simulink model "LKAS_AutoSave_20210315_1628"  (R2018b)
settings: Solver=FixedStepDiscrete  StartTime=0.0  StopTime=10.0  FixedStep=0.01  RelTol=1e-3
InitFcn:
  | tmpVer = ver('MATLAB');
  | tmpVer = str2num(tmpVer.Version);
  | % -------------------------------------------------------------------
  | %  MATLAB file generated by Simulink.saveVars on 21-Nov-2019 10:06:14
  | %  MATLAB version: 7.13.0.564 (R2011b)
  | % -------------------------------------------------------------------
  | 
  | 
  | SInt16 = Simulink.AliasType;
  | SInt16.Description = 'Num';
  | if (tmpVer > 7.11)
  | 	SInt16.DataScope = 'Auto';
  | end
  | SInt16.HeaderFile = 'Rte_Type.h';
  | SInt16.BaseType = 'int16';
  | 
  | SInt32 = Simulink.AliasType;
  | SInt32.Description = 'Num';
  | if (tmpVer > 7.11)
  | 	SInt32.DataScope = 'Auto';
  | end
  | SInt32.HeaderFile = 'Rte_Type.h';
  | SInt32.BaseType = 'int32';
  | 
  | SInt8 = Simulink.AliasType;
  | SInt8.Description = 'Num';
  | if (tmpVer > 7.11)
  | 	SInt8.DataScope = 'Auto';
  | end
  | SInt8.HeaderFile = 'Rte_Type.h';
  | SInt8.BaseType = 'int8';
  | 
  | T_A_m2_1024_1_u32 = Simulink.NumericType;
  | T_A_m2_1024_1_u32.Description = 'm2 (square meters  (m2))';
  | if (tmpVer > 7.11)
  | 	T_A_m2_1024_1_u32.DataScope = 'Auto';
  | end
  | T_A_m2_1024_1_u32.HeaderFile = 'Rte_Type.h';
  | T_A_m2_1024_1_u32.DataTypeMode = 'Fixed-point: slope and bias scaling';
  | T_A_m2_1024_1_u32.SignednessBool = false;
  | T_A_m2_1024_1_u32.WordLength = 32;
  | T_A_m2_1024_1_u32.FixedExponent = -10;
  | T_A_m2_1024_1_u32.SlopeAdjustmentFactor = 1;
  | T_A_m2_1024_1_u32.Bias = 0;
  | T_A_m2_1024_1_u32.DataTypeOverride = 'Inherit';
  | T_A_m2_1024_1_u32.IsAlias = true;
  | 
  | T_A_m2_65536_1_u16 = Simulink.NumericType;
  | T_A_m2_65536_1_u16.Description = 'm2 (square meters  (m2))';
  | if (tmpVer > 7.11)
  | 	T_A_m2_65536_1_u16.DataScope = 'Auto';
  | end
  | T_A_m2_65536_1_u16.HeaderFile = 'Rte_Type.h';
  | T_A_m2_65536_1_u16.DataTypeMode = 'Fixed-point: slope and bias scaling';
  | T_A_m2_65536_1_u16.SignednessBool = false;
  | T_A_m2_65536_1_u16.WordLength = 16;
  | T_A_m2_65536_1_u16.FixedExponent = -16;
  | T_A_m2_65536_1_u16.SlopeAdjustmentFactor = 1;
  | T_A_m2_65536_1_u16.Bias = 0;
  | T_A_m2_65536_1_u16.DataTypeOverride = 'Inherit';
  | ... (+4598 lines)
StopFcn:
  | clear  T_A_m2_1024_1_u32 T_A_m2_65536_1_u16 T_A_m2_Float32 T_A_mm2_10_1_u16 T_A_mm2_4_1_s16 T_A_mm2_Float32 T_Cnt_Num_10_1_u32 T_Cnt_Num_1_1_s16 T_Cnt_Num_1_1_s32 T_Cnt_Num_1_1_s8 T_Cnt_Num_1_1_u16 T_Cnt_Num_1_1_u32 T_Cnt_Num_1_1_u8 T_E_J_1_1_s32 T_E_J_Float32 T_E_kJ_128_1_s32 T_E_kJ_Float32 T_E_kwh_10_1_u16 T_E_kwh_Float32 T_Epl_kwhpkm_100_1_u16 T_Epl_kwhpkm_Float32 T_F_N_1_1_s16 T_F_N_Float32 T_I_A_1000_1_u16 T_I_A_1048576_1_s32 T_I_A_2048_1_s16 T_I_A_32_1_s16 T_I_A_Float32 T_I_mA_1_1_s16 T_I_mA_32768_128_s16 T_I_mA_Float32 T_J_kgpm2_128_1_u16 T_J_kgpm2_Float32 T_K_NA_1000_1_s16 T_K_NA_100_1_s16 T_K_NA_100_1_u16 T_K_NA_1024_1_s16 T_K_NA_1024_1_u16 T_K_NA_128_1_s16 T_K_NA_128_1_u16 T_K_NA_128_1_u8 T_K_NA_16777216_1_u32 T_K_NA_16_1_s16 T_K_NA_16_1_u16 T_K_NA_16_1_u8 T_K_NA_1_16_u16 T_K_NA_1_1_s16 T_K_NA_1_1_u16 T_K_NA_1_1_u8 T_K_NA_32768_1_s16 T_K_NA_32768_1_u16 T_K_NA_32_1_s8 T_K_NA_4096_1_u16 T_K_NA_4194304_1_s32 T_K_NA_4194304_1_u16 T_K_NA_65536_1_s32 T_K_NA_65536_1_u16 T_K_NA_8192_1_s16 T_K_NA_8_1_s16 T_K_NA_Float32 T_M_Nm_16_1_s16 T_M_Nm_1_1_s16 T_M_Nm_32768_1_s16 T_M_Nm_32_1_s16 T_M_Nm_4_1_s16 T_M_Nm_512_1_s16 T_M_Nm_Float32 T_P_W_1_4_s16 T_P_W_1_8_s16 T_P_W_Float32 T_P_kW_128_1_s16 T_P_kW_1_8_s16 T_P_kW_8_1_s32 T_P_kW_Float32 T_Pct_pct_1024_1_s32 T_Pct_pct_1024_1_u32 T_Pct_pct_10_1_s16 T_Pct_pct_10_1_u32 T_Pct_pct_128_100_s8 T_Pct_pct_1_1_s16 T_Pct_pct_1_4_u8 T_Pct_pct_255_100_u16 T_Pct_pct_255_100_u8 T_Pct_pct_256_1_s16 T_Pct_pct_256_1_u16 T_Pct_pct_65535_100_u16 T_Pct_pct_Float32 T_R_ohm_1024_1_s16 T_R_ohm_32_1_s16 T_R_ohm_Float32 T_TK_K_16_1_s16 T_TK_K_Float32 T_T_degC_10_400_1_u16 T_T_degC_16_1_s16 T_T_degC_1_40_1_u8 T_T_degC_2_80_1_u8 T_T_degC_Float32 T_U_V_1000_1_u16 T_U_V_10_1_u8 T_U_V_200_1_u8 T_U_V_32_1_s16 T_U_V_4096_1_s16 T_U_V_512_1_s16 T_U_V_65535_8_u16 T_U_V_8192_1_u16 T_U_V_Float32 T_U_mV_1_1_s16 T_U_mV_256_20_u16 T_U_mV_Float32 T_V_l_256_1_s16 T_V_l_4096_1_s16 T_V_l_64_1_s16 T_V_l_65535_100_u16 T_V_l_Float32 T_V_ml_128_1_s16 T_V_ml_1_1_s16 T_V_ml_32768_1_s16 T_V_ml_Float32 T_V_ul_32_1_u16 T_V_ul_Float32 T_Vpl_clpkm_512_1_u16 T_Vpl_clpkm_Float32 T_a_kphps_16_1_s16 T_a_kphps_Float32 T_a_mps2_128_1_s16 T_a_mps2_Float32 T_c_MJpkg_256_1_s16 T_c_MJpkg_Float32 T_c_kJpgpK_1024_1_s16 T_c_kJpgpK_Float32 T_c_kJpkgpK_128_1_u16 T_c_kJpkgpK_Float32 T_chrg_Ah_1_1_s16 T_chrg_Ah_1_1_u16 T_chrg_Ah_1_1_u8 T_chrg_Ah_256_1_u16 T_chrg_Ah_4194304_1_s32 T_chrg_Ah_512_1_u16 T_chrg_Ah_8_1_u16 T_chrg_Ah_Float32 T_cmp_NA_100_1_s16 T_cmp_NA_128_1_s16 T_cmp_NA_16_1_s16 T_cmp_NA_32768_1_u16 T_cmp_NA_Float32 T_d2n_rpmps2_4_1_s16 T_d2n_rpmps2_Float32 T_dPct_pctps_16_1_s16 T_dPct_pctps_256_1_s16 T_dPct_pctps_Float32 T_dT_degCps_128_1_s16 T_dT_degCps_Float32 T_dV_lph_1_1_s16 T_dV_lph_Float32 T_dV_lpm_128_1_s16 T_dV_lpm_32_1_s16 T_dV_lpm_Float32 T_dV_lps_1024_1_u16 T_dV_lps_4_1_u16 T_dV_lps_Float32 T_dV_mlps_1024_1_s16 T_dV_mlps_Float32 T_d_BitField16 T_dm_gps_128_1_s16 T_dm_gps_128_1_u16 T_dm_gps_256_1_u16 T_dm_gps_Float32 T_dm_mgps_1_1_s16 T_dm_mgps_Float32 T_dn_rpmps_1_1_s16 T_dn_rpmps_2_1_s16 T_dn_rpmps_Float32 T_dp_Paps_1_1_s16 T_dp_Paps_Float32 T_dp_kPaps_1_1_s16 T_dp_kPaps_8_1_s16 T_dp_kPaps_Float32 T_dphi_degps_128_1_s16 T_dphi_degps_8_1_s16 T_dphi_degps_Float32 T_dr_ps_256_1_s16 T_dr_ps_Float32 T_drho_mgplps_1_2_s16 T_drho_mgplps_Float32 T_e_NA_1_1_u8 T_f_Hz_1_1_u16 T_f_Hz_1_1_u32 T_f_Hz_64_1_u16 T_f_Hz_8_1_s16 T_f_Hz_Float32 T_g_BitField32 T_l_km_16_1_s16 T_l_km_1_1_u16 T_l_km_1_1_u32 T_l_km_Float32 T_l_m_1024_1_s16 T_l_m_16_1_s16 T_l_m_1_1_u32 T_l_m_Float32 T_l_mm_16_1_s16 T_l_mm_1_1_u16 T_l_mm_4096_1_s16 T_l_mm_4_1_u8 T_l_mm_64_1_s16 T_l_mm_Float32 T_m_g_1_1_s16 T_m_g_2048_1_s16 T_m_g_32_1_u16 T_m_g_Float32 T_m_kg_1024_1_s16 T_m_kg_1_1_s16 T_m_kg_1_1_u32 T_m_kg_Float32 T_m_mg_128_1_s16 T_m_mg_32_1_s16 T_m_mg_Float32 T_n_rpm_1_1_s16 T_n_rpm_1_25_u8 T_n_rpm_256_50_u16 T_n_rpm_2_25_u8 T_n_rpm_4_1_u16 T_n_rpm_Float32 T_p_MPa_64_1_s16 T_p_MPa_Float32 T_p_Pa_1_1_s16 T_p_Pa_Float32 T_p_kPa_1_10_u16 T_p_kPa_1_1_s16 T_p_kPa_1_1_u8 T_p_kPa_256_1_u16 T_p_kPa_32_1_u16 T_p_kPa_64_1_s16 T_p_kPa_Float32 T_phi_deg_100_1_s16 T_phi_deg_1024_1_s16 T_phi_deg_128_1_s16 T_phi_deg_1_1_u8 T_phi_deg_256_1_s16 T_phi_deg_2_1_s8 T_phi_deg_32_1_s16 T_phi_deg_512_6_s32 T_phi_deg_Float32 T_phi_rad_2048_1_s16 T_phi_rad_Float32 T_r_NA_1024_1_s16 T_r_NA_1024_1_u16 T_r_NA_16384_1_s16 T_r_NA_16_1_s16 T_r_NA_256_1_s8 T_r_NA_256_1_u16 T_r_NA_32768_1_u16 T_r_NA_32_1_u16 T_r_NA_4096_1_s16 T_r_NA_65535_2_u16 T_r_NA_8192_1_u16 T_r_NA_Float32 T_rho_gpl_8192_1_s16 T_rho_gpl_Float32 T_rho_kgpm3_16_1_s16 T_rho_kgpm3_Float32 T_rho_mgpl_1_1_s16 T_rho_mgpl_64_1_s16 T_rho_mgpl_Float32 T_t_hour_1_1_s16 T_t_hour_Float32 T_t_m_1_1_u16 T_t_m_Float32 T_t_ms_1_1_s16 T_t_ms_1_1_u16 T_t_ms_1_1_u32 T_t_ms_4096_1_s16 T_t_ms_64_1_s16 T_t_ms_Float32 T_t_s_1000_1_s16 T_t_s_100_1_s16 T_t_s_10_1_s16 T_t_s_10_1_u16 T_t_s_1_1_s16 T_t_s_1_1_u16 T_t_s_1_1_u32 T_t_s_Float32 T_t_us_10_1_u32 T_t_us_1_1_s16 T_t_us_1_1_u32 T_t_us_1_4_u16 T_t_us_Float32 T_v_kph_1_1_u8 T_v_kph_64_1_s16 T_v_kph_64_1_u16 T_v_kph_Float32 T_v_mps_256_1_s16 T_v_mps_Float32 T_w_radps_32_1_s16 T_w_radps_Float32 T_y_BitField8 T_y_BitFieldDiagProgress T_y_BitFieldDiagStatus T_y_NA_1_1_u8 SInt16 SInt32 SInt8 T_BOOLEAN UInt16 UInt32 UInt8 s16 s32 s8 u16 u32 u8
model workspace (MAT data in the model file):
  MCOS : class17 (value not decoded)
  MCOS : class17 (value not decoded)
  MCOS : class17 (value not decoded)
  MCOS : class17 (value not decoded)
  MCOS : class17 (value not decoded)
  MCOS : class17 (value not decoded)
  MCOS : class17 (value not decoded)
  MCOS : class17 (value not decoded)
  MCOS : class17 (value not decoded)
  MCOS : class17 (value not decoded)
  MCOS : class17 (value not decoded)
  MCOS : class17 (value not decoded)
  MCOS : class17 (value not decoded)
  MCOS : class17 (value not decoded)
  MCOS : class17 (value not decoded)
  MCOS : class17 (value not decoded)
  MCOS : class17 (value not decoded)
  MCOS : class17 (value not decoded)
  MCOS : class17 (value not decoded)
  MCOS : class17 (value not decoded)
  MCOS : class17 (value not decoded)
  MCOS : class17 (value not decoded)
  MCOS : class17 (value not decoded)
  MCOS : class17 (value not decoded)
  MCOS : class17 (value not decoded)
  MCOS : class17 (value not decoded)
  MCOS : class17 (value not decoded)
  MCOS : class17 (value not decoded)
  MCOS : class17 (value not decoded)
  MCOS : class17 (value not decoded)
  MCOS : class17 (value not decoded)
  MCOS : class17 (value not decoded)
  MCOS : class17 (value not decoded)
  MCOS : class17 (value not decoded)
  MCOS : class17 (value not decoded)
  MCOS : class17 (value not decoded)
  MCOS : class17 (value not decoded)
  MCOS : class17 (value not decoded)
  MCOS : class17 (value not decoded)
  MCOS : class17 (value not decoded)
  MCOS : class17 (value not decoded)
  MCOS : class17 (value not decoded)
  MCOS : class17 (value not decoded)
  MCOS : class17 (value not decoded)
  MCOS : class17 (value not decoded)
  MCOS : class17 (value not decoded)
  MCOS : class17 (value not decoded)
  MCOS : class17 (value not decoded)
  MCOS : class17 (value not decoded)
  MCOS : class17 (value not decoded)
  MCOS : class17 (value not decoded)
  MCOS : class17 (value not decoded)
  MCOS : class17 (value not decoded)
  MCOS : class17 (value not decoded)
  MCOS : class17 (value not decoded)
  MCOS : class17 (value not decoded)
  MCOS : class17 (value not decoded)
  MCOS : class17 (value not decoded)
  MCOS : class17 (value not decoded)
  MCOS : class17 (value not decoded)
  MCOS : class17 (value not decoded)
  MCOS : class17 (value not decoded)
  MCOS : class17 (value not decoded)
  MCOS : class17 (value not decoded)
  MCOS : class17 (value not decoded)
  MCOS : class17 (value not decoded)
  MCOS : class17 (value not decoded)
  MCOS : class17 (value not decoded)
  MCOS : class17 (value not decoded)
  MCOS : class17 (value not decoded)
  MCOS : class17 (value not decoded)
  MCOS : class17 (value not decoded)
  MCOS : class17 (value not decoded)
  MCOS : class17 (value not decoded)
  MCOS : class17 (value not decoded)
  MCOS : class17 (value not decoded)
  MCOS : class17 (value not decoded)
  MCOS : class17 (value not decoded)
  MCOS : class17 (value not decoded)
  MCOS : class17 (value not decoded)
  MCOS : class17 (value not decoded)
  MCOS : class17 (value not decoded)
  MCOS : class17 (value not decoded)
  MCOS : class17 (value not decoded)
  MCOS : class17 (value not decoded)
  MCOS : class17 (value not decoded)
  MCOS : class17 (value not decoded)
  MCOS : class17 (value not decoded)
  MCOS : class17 (value not decoded)
  MCOS : class17 (value not decoded)
  MCOS : class17 (value not decoded)
  MCOS : class17 (value not decoded)
  MCOS : class17 (value not decoded)
  MCOS : class17 (value not decoded)
undefined symbols (not defined in the file): LKA_CarWidth, LKA_SampleTime, LKA_StrRatio_C, LKA_Veh2CamL_C, LKA_Veh2CamW_C, LKA_WhlBaseL_C, LL_CompSWA_C, LL_CrvtPrvwT_C, LL_DesDvt_C, LL_DvtComp_C, LL_DvtPrvwT_C, LL_DvtSpdDet_vDvtSpdMin_C, LL_HdAgExT_C, LL_HdAgPrvwT_C, LL_LAccMax_C, LL_LAccRMax_C, LL_LDW_EarliestWarnLine_C, LL_LDW_LatestWarnLine_C, LL_LDWS_SUPPRESS_HEADING, LL_LFClb_TFC_DiffCtlBalance, LL_LFClb_TFC_DiffCtrlMaxSWA, LL_LFClb_TFC_DiffCtrlRatio, LL_LFClb_TFC_facmGainLutGain1_C, LL_LFClb_TFC_facmGainLutGain2_C, LL_LFClb_TFC_facmIntegRatio, LL_LFClb_TFC_facmKlat_C, LL_LFClb_TFC_FfCtlRatio_C, LL_LFClb_TFC_phiIntegCtlMaxSWA_C, LL_LFClb_TFC_tiKlatPrvwT_C, LL_LFClb_TFC_vGainLutVehSpdLwr_C, LL_LFClb_TFC_vGainLutVehSpdUpr_C, LL_LKA_EarliestWarnLine_C, LL_LKA_LatestWarnLine_C, LL_LKAExPrcs_ExitC0Dvt, LL_LKAExPrcs_ExitC0Swt, LL_LKAExPrcs_tiExitTime1, LL_LKAExPrcs_tiExitTime2, LL_LKAExPrcs_tiExitTime3, LL_LKAS_OUT_OF_CONTROL_LAT_VEL, LL_LKAS_OUT_OF_CONTROL_TTLC, LL_LKASWASyn_M0, LL_LKASWASyn_M1, LL_LKASWASyn_M2, LL_LKASWASyn_M3K, LL_LKASWASyn_SWAaddMax, LL_LKASWASyn_T2, LL_LKASWASyn_tiTrqSwaRtTime, LL_LKASWASyn_tiTrqSwaTime, LL_LKASWASyn_TrqMax, LL_LKASWASyn_TrqSwaAddSwt, LL_LKASWASyn_TrqSwaRateDiff, LL_LSpdCompT_C, LL_lStpLngth_C, LL_MAX_DELAY_EPSSTAR_TIME, LL_MAX_DRIVER_TORQUE_DISABLE, LL_MAX_DRIVER_TORQUE_ENABLE, LL_MAX_LANE_WIDTH_DISABLE, LL_MAX_LANE_WIDTH_ENABLE, LL_MAX_LAT_ACC_DISABLE, LL_MAX_LAT_ACC_ENABLE ... (+34)
libraries: simulink x130, dspstat3 x3, simulink_extras x1
(part 16 of 18)

== system LKAS_AutoSave_20210315_1628/LKAS/LL/LLOn/LL State Determination (LLStateDet)/LL State Machine Conditions (LLSMCon)/Enable Condition (EnaC)/LKA Own Condition (LKAOwnC)/EPS State Condition (EPSStC) ==
  EPSStC_bsEPSInfo : Inport
  Bus Selector : BusSelector  OutputSignals=EPS_LKA_State
  Compare To Constant1 : simulink/Logic and Bit Operations/Compare To Constant  relop===  const=2  OutDataTypeStr=boolean
  Compare To Constant2 : simulink/Logic and Bit Operations/Compare To Constant  relop===  const=1  OutDataTypeStr=boolean
  Logical Operator : Logic  Operator=OR  AllPortsSameDT=off  OutDataTypeStr=boolean
  EPSStC_tfEPSCtlEC : Outport
  wires:
  EPSStC_bsEPSInfo/1 -> Bus Selector/1
  Logical Operator/1 -> EPSStC_tfEPSCtlEC/1
  Bus Selector/1 -> Compare To Constant2/1, Compare To Constant1/1  "<EPS_LKA_State>"
  Compare To Constant1/1 -> Logical Operator/1
  Compare To Constant2/1 -> Logical Operator/2

== system LKAS_AutoSave_20210315_1628/LKAS/LL/LLOn/LL State Determination (LLStateDet)/LL State Machine Conditions (LLSMCon)/Enable Condition (EnaC)/LKA Own Condition (LKAOwnC)/Exit Lane Delay (ExLaneDel) ==
  ExLaneDel_stVehExLane : Inport
  ExLaneDel_tiExLaneDelT : Inport  Port=2
  Bus Selector2 : BusSelector  OutputSignals=LKA_SampleTime
  Cast To Single1 : DataTypeConversion  OutDataTypeStr=uint16
  Compare To Zero : simulink/Logic and Bit Operations/Compare To Zero  relop===  OutDataTypeStr=boolean
  Detect Fall Nonpositive : simulink/Logic and Bit Operations/Detect Fall Nonpositive  vinit=0  OutDataTypeStr=boolean
      settings: SourceProductName=Simulink  SourceProductBaseCode=SL
  Detect Rise Positive1 : simulink/Logic and Bit Operations/Detect Rise Positive  vinit=0  OutDataTypeStr=boolean
  Divide : Product  Inputs=*/
  If Action Subsystem3 : Subsystem  TreatAsAtomicUnit=on
  If Action Subsystem4 : Subsystem  TreatAsAtomicUnit=on
  If Action Subsystem5 : Subsystem  TreatAsAtomicUnit=on
  If1 : If  NumInputs=4  IfExpression=u1 == 1 & u2 == 1  ElseIfExpressions=u3 == 0 & u4 == 1
  Memory1 : Memory  InheritSampleTime=on
  Memory2 : Memory  InheritSampleTime=on
  Merge : Merge  Inputs=3
  Sum Condition1 : Subsystem  TreatAsAtomicUnit=on
  ExLaneDel_stExLaneDel : Outport
  wires:
  Merge/1 -> Memory1/1, Sum Condition1/1(In), Sum Condition1/Enable, Compare To Zero/1
  Memory1/1 -> If Action Subsystem5/1(In1)
  Memory2/1 -> Detect Fall Nonpositive/1, If1/3
  ExLaneDel_tiExLaneDelT/1 -> Divide/1
  If1/2 -> If Action Subsystem4/Action
  If1/1 -> If Action Subsystem3/Action
  If1/3 -> If Action Subsystem5/Action
  Detect Rise Positive1/1 -> If1/2
  ExLaneDel_stVehExLane/1 -> If1/1, Detect Rise Positive1/1
  Detect Fall Nonpositive/1 -> If1/4
  If Action Subsystem3/1(Out) -> Merge/1
  If Action Subsystem5/1(Out) -> Merge/3
  If Action Subsystem4/1(Out) -> Merge/2
  Sum Condition1/1(Out) -> Memory2/1
  Compare To Zero/1 -> ExLaneDel_stExLaneDel/1
  Divide/1 -> Cast To Single1/1
  Bus Selector2/1 -> Divide/2  "<LKA_SampleTime>"
  [LLClb_bsConstantClb] -> Bus Selector2/1
  Cast To Single1/1 -> Sum Condition1/2(Sum)

== system LKAS_AutoSave_20210315_1628/LKAS/LL/LLOn/LL State Determination (LLStateDet)/LL State Machine Conditions (LLSMCon)/Enable Condition (EnaC)/LKA Own Condition (LKAOwnC)/LKA Own Condition Synthesis (LKAOwnCSyn) ==
  LKAOwnCSyn_stDACMode : Inport
  LKAOwnCSyn_stEPSCtlEC : Inport  Port=2
  LKAOwnCSyn_stVehLSpdC : Inport  Port=3
  LKAOwnCSyn_stVehPosChk : Inport  Port=4
  LKAOwnCSyn_stExLaneDel : Inport  Port=5
  Compare To Constant : simulink/Logic and Bit Operations/Compare To Constant  relop===  const=2  OutDataTypeStr=boolean
  Compare To Constant{1..2,4..5} (4 alike) : simulink/Logic and Bit Operations/Compare To Constant  relop===  const=1  OutDataTypeStr=boolean
  Logical Operator : Logic  Inputs=4  AllPortsSameDT=off  OutDataTypeStr=boolean
  LKAOwnCSyn_stLKAPptyCSyn : Outport
  wires:
  LKAOwnCSyn_stDACMode/1 -> Compare To Constant/1
  LKAOwnCSyn_stVehPosChk/1 -> Compare To Constant1/1
  Logical Operator/1 -> LKAOwnCSyn_stLKAPptyCSyn/1
  LKAOwnCSyn_stEPSCtlEC/1 -> Compare To Constant2/1
  LKAOwnCSyn_stExLaneDel/1 -> Compare To Constant5/1
  Compare To Constant/1 -> Logical Operator/1
  Compare To Constant2/1 -> Logical Operator/2
  Compare To Constant4/1 -> Logical Operator/3
  Compare To Constant1/1 -> Logical Operator/4
  Compare To Constant5/1 -> ?
  LKAOwnCSyn_stVehLSpdC/1 -> Compare To Constant4/1

== system LKAS_AutoSave_20210315_1628/LKAS/LL/LLOn/LL State Determination (LLStateDet)/LL State Machine Conditions (LLSMCon)/Enable Condition (EnaC)/LKA Own Condition (LKAOwnC)/Vehicle Lateral Speed Condition (VehLSpdC) ==
  VehLSpdC_bsTTLCInfo : Inport
  VehLSpdC_vVehLSpdMax_C : Inport  Port=2
  Abs1 : Abs
  Abs2 : Abs
  Bus Selector2 : BusSelector  OutputSignals=vLft,vRgt
  Logical Operator : Logic  AllPortsSameDT=off  OutDataTypeStr=boolean
  Relational Operator2 : RelationalOperator  Operator=<=  OutDataTypeStr=boolean  RndMeth=Nearest
  Relational Operator3 : RelationalOperator  Operator=<=  OutDataTypeStr=boolean  RndMeth=Nearest
  VehLSpdC_stVehLSpdC : Outport
  wires:
  VehLSpdC_vVehLSpdMax_C/1 -> Relational Operator3/2, Relational Operator2/2
  Abs1/1 -> Relational Operator2/1
  Relational Operator2/1 -> Logical Operator/1
  Abs2/1 -> Relational Operator3/1
  Bus Selector2/1 -> Abs1/1  "<vLft>"
  Bus Selector2/2 -> Abs2/1  "<vRgt>"
  VehLSpdC_bsTTLCInfo/1 -> Bus Selector2/1
  Logical Operator/1 -> VehLSpdC_stVehLSpdC/1
  Relational Operator3/1 -> Logical Operator/2

== system LKAS_AutoSave_20210315_1628/LKAS/LL/LLOn/LL State Determination (LLStateDet)/LL State Machine Conditions (LLSMCon)/Enable Condition (EnaC)/LKA Own Condition (LKAOwnC)/Vehicle Position Check (VehPosChk)1 ==
  VehPosChk_LaneWidth : Inport
  VehPosChk_bsDvtInfo : Inport  Port=2
  VehPosChk_lWarnLineMax_C : Inport  Port=3
  VehPosChk_lWarnLineMin_C : Inport  Port=4
  Bus Selector : BusSelector  OutputSignals=ILftDvt,IRgtDvt
  Logical Operator : Logic  AllPortsSameDT=off  OutDataTypeStr=boolean
  Logical Operator1 : Logic  Operator=OR  AllPortsSameDT=off  OutDataTypeStr=boolean
  Relational Operator1 : RelationalOperator  OutDataTypeStr=boolean  RndMeth=Nearest
  Relational Operator2 : RelationalOperator  OutDataTypeStr=boolean  RndMeth=Nearest
  Relational Operator3 : RelationalOperator  Operator=<=  OutDataTypeStr=boolean  RndMeth=Nearest
  Relational Operator4 : RelationalOperator  Operator=<=  OutDataTypeStr=boolean  RndMeth=Nearest
  Subsystem : Subsystem
  VehPosChk_stVehPosChk : Outport
  VehPosChk_stVehExLane : Outport  Port=2
  wires:
  Bus Selector/1 -> Relational Operator4/1, Relational Operator1/1  "<ILftDvt>"
  Bus Selector/2 -> Relational Operator2/1, Relational Operator3/1  "<IRgtDvt>"
  Relational Operator1/1 -> Logical Operator/1
  Relational Operator2/1 -> Logical Operator/2
  Logical Operator/1 -> VehPosChk_stVehPosChk/1
  VehPosChk_bsDvtInfo/1 -> Bus Selector/1
  Subsystem/1(EnableLine) -> Relational Operator1/2, Relational Operator2/2
  VehPosChk_lWarnLineMax_C/1 -> Subsystem/1(WarnLine_C)
  VehPosChk_LaneWidth/1 -> Subsystem/2(LaneWidth)
  Logical Operator1/1 -> VehPosChk_stVehExLane/1
  Relational Operator3/1 -> Logical Operator1/2
  VehPosChk_lWarnLineMin_C/1 -> Relational Operator3/2, Relational Operator4/2
  Relational Operator4/1 -> Logical Operator1/1

== system LKAS_AutoSave_20210315_1628/LKAS/LL/LLOn/LL State Determination (LLStateDet)/LL State Machine Conditions (LLSMCon)/Enable Condition (EnaC)/Lane Condition (LaneC)/Lane C1 Detection (LaneC1Det) ==
  LaneWDet_facmL0C1 : Inport
  LaneWDet_facmR0C1 : Inport  Port=2
  Abs : Abs
  Add : Sum  Inputs=+-  OutDataTypeStr=single
  Compare To Constant1 : simulink/Logic and Bit Operations/Compare To Constant  relop=<=  const=0.025  OutDataTypeStr=boolean
  LaneC1Det_stLaneC1DetFlg : Outport
  wires:
  LaneWDet_facmR0C1/1 -> Add/2
  LaneWDet_facmL0C1/1 -> Add/1
  Add/1 -> Abs/1
  Compare To Constant1/1 -> LaneC1Det_stLaneC1DetFlg/1
  Abs/1 -> Compare To Constant1/1

== system LKAS_AutoSave_20210315_1628/LKAS/LL/LLOn/LL State Determination (LLStateDet)/LL State Machine Conditions (LLSMCon)/Enable Condition (EnaC)/Lane Condition (LaneC)/Lane Condition Synthesis (LaneCSyn) ==
  LaneCSyn_stLaneQlECFlg : Inport
  LaneCSyn_stLaneWDetFlg : Inport  Port=2
  LaneCSyn_stLaneCrvtDetFlg : Inport  Port=3
  LaneCSyn_stLaneC1DetFlg : Inport  Port=4
  Logical Operator3 : Logic  Inputs=4  AllPortsSameDT=off  OutDataTypeStr=boolean
  LaneCSyn_stLaneCSyn : Outport
  wires:
  LaneCSyn_stLaneQlECFlg/1 -> Logical Operator3/1
  LaneCSyn_stLaneCrvtDetFlg/1 -> Logical Operator3/3
  Logical Operator3/1 -> LaneCSyn_stLaneCSyn/1
  LaneCSyn_stLaneWDetFlg/1 -> Logical Operator3/2
  LaneCSyn_stLaneC1DetFlg/1 -> Logical Operator3/4

== system LKAS_AutoSave_20210315_1628/LKAS/LL/LLOn/LL State Determination (LLStateDet)/LL State Machine Conditions (LLSMCon)/Enable Condition (EnaC)/Lane Condition (LaneC)/Lane Curvature Detection (LaneCrvtDet) ==
  LaneCrvtDet_crPrvwCrvt : Inport
  LaneCrvtDet_crLaneCrvtMax_C : Inport  Port=2
  Abs : Abs
  Constant : Constant  Value=0  OutDataTypeStr=single  SampleTime=-1
  Interval Test Dynamic : simulink/Logic and Bit Operations/Interval Test Dynamic  IntervalClosedRight=on  IntervalClosedLeft=on  OutDataTypeStr=boolean
      settings: SourceProductName=Simulink  SourceProductBaseCode=SL
  LaneCrvtDet_stLaneCrvtDetFlg : Outport
  wires:
  Interval Test Dynamic/1 -> LaneCrvtDet_stLaneCrvtDetFlg/1
  LaneCrvtDet_crLaneCrvtMax_C/1 -> Interval Test Dynamic/1
  Constant/1 -> Interval Test Dynamic/3
  LaneCrvtDet_crPrvwCrvt/1 -> Abs/1
  Abs/1 -> Interval Test Dynamic/2

== system LKAS_AutoSave_20210315_1628/LKAS/LL/LLOn/LL State Determination (LLStateDet)/LL State Machine Conditions (LLSMCon)/Enable Condition (EnaC)/Lane Condition (LaneC)/Lane Quality Enable Condition (LaneQlEC) ==
  LaneQlEC_stFacmL0Ql : Inport
  LaneQlEC_stFacmR0Ql : Inport  Port=2
  Compare To Constant : simulink/Logic and Bit Operations/Compare To Constant  relop=>  const=2  OutDataTypeStr=boolean
  Compare To Constant1 : simulink/Logic and Bit Operations/Compare To Constant  relop=>  const=2  OutDataTypeStr=boolean
  Logical Operator : Logic  AllPortsSameDT=off  OutDataTypeStr=boolean
  LaneQlEC_stLaneQlECFlg : Outport
  wires:
  LaneQlEC_stFacmL0Ql/1 -> Compare To Constant/1
  LaneQlEC_stFacmR0Ql/1 -> Compare To Constant1/1
  Compare To Constant/1 -> Logical Operator/1
  Compare To Constant1/1 -> Logical Operator/2
  Logical Operator/1 -> LaneQlEC_stLaneQlECFlg/1

== system LKAS_AutoSave_20210315_1628/LKAS/LL/LLOn/LL State Determination (LLStateDet)/LL State Machine Conditions (LLSMCon)/Enable Condition (EnaC)/Lane Condition (LaneC)/Lane Width Detection (LaneWDet) ==
  LaneWDet_LaneWidth : Inport
  LaneWDet_lLaneWMax : Inport  Port=2
  LaneWDet_lLaneWMin : Inport  Port=3
  Abs1 : Abs
  Interval Test Dynamic : simulink/Logic and Bit Operations/Interval Test Dynamic  IntervalClosedRight=on  IntervalClosedLeft=on  OutDataTypeStr=boolean
      settings: SourceProductName=Simulink  SourceProductBaseCode=SL
  LaneWDet_stLaneWDetFlg : Outport
  wires:
  Interval Test Dynamic/1 -> LaneWDet_stLaneWDetFlg/1
  LaneWDet_lLaneWMax/1 -> Interval Test Dynamic/1
  LaneWDet_lLaneWMin/1 -> Interval Test Dynamic/3
  Abs1/1 -> Interval Test Dynamic/2
  LaneWDet_LaneWidth/1 -> Abs1/1

== system LKAS_AutoSave_20210315_1628/LKAS/LL/LLOn/LL State Determination (LLStateDet)/LL State Machine Conditions (LLSMCon)/Enable Condition (EnaC)/Vehicle State Condition (VehStateC)/Emergency Light Enable Condition (EmgcyLghtEC) ==
  EmgcyLghtEC_bsStLampState : Inport
  Add : Sum
  Bus Selector : BusSelector  OutputSignals=BCM_Double_Light,BCM_Left_Light,BCM_Right_Light
  Compare To Constant : simulink/Logic and Bit Operations/Compare To Constant  relop=<=  const=0  OutDataTypeStr=boolean
  Compare To Constant1 : simulink/Logic and Bit Operations/Compare To Constant  relop=>  const=0  OutDataTypeStr=boolean
  Compare To Constant2 : simulink/Logic and Bit Operations/Compare To Constant  relop=>  const=0  OutDataTypeStr=boolean
  Compare To Constant3 : simulink/Logic and Bit Operations/Compare To Constant  relop=>  const=0  OutDataTypeStr=boolean
  Constant : Constant  Value=3  OutDataTypeStr=single
  Constant1 : Constant  Value=-1  OutDataTypeStr=single
  Logical Operator : Logic  Operator=OR  Inputs=3  AllPortsSameDT=off  OutDataTypeStr=boolean
  Memory : Memory  InheritSampleTime=on
  Saturation : Saturate  UpperLimit=200  LowerLimit=-1
      settings: AttributesFormatString="Min = %<LowerLimit>  Max = %<UpperLimit>"
  Switch : Switch  Criteria=u2 > Threshold
  EmgcyLghtEC_stEmgcyLghtECFlg : Outport
  wires:
  Compare To Constant2/1 -> Logical Operator/2
  Compare To Constant1/1 -> Logical Operator/1
  EmgcyLghtEC_bsStLampState/1 -> Bus Selector/1
  Bus Selector/1 -> Compare To Constant1/1  "<BCM_Double_Light>"
  Bus Selector/2 -> Compare To Constant2/1  "<BCM_Left_Light>"
  Logical Operator/1 -> Switch/2
  Constant/1 -> Switch/1
  Constant1/1 -> Switch/3
  Switch/1 -> Add/1
  Add/1 -> Saturation/1
  Saturation/1 -> Compare To Constant/1, Memory/1
  Memory/1 -> Add/2
  Compare To Constant/1 -> EmgcyLghtEC_stEmgcyLghtECFlg/1
  Bus Selector/3 -> Compare To Constant3/1  "<BCM_Right_Light>"
  Compare To Constant3/1 -> Logical Operator/3

== system LKAS_AutoSave_20210315_1628/LKAS/LL/LLOn/LL State Determination (LLStateDet)/LL State Machine Conditions (LLSMCon)/Enable Condition (EnaC)/Vehicle State Condition (VehStateC)/Gear Enable Condition (GearEC) ==
  GearEC_bsTCUState : Inport
  Bus Selector : BusSelector  OutputSignals=TCU_ActualGear
  Compare To Constant : simulink/Logic and Bit Operations/Compare To Constant  relop===  const=3  OutDataTypeStr=boolean
  GearEC_stGearECFlg : Outport
  wires:
  GearEC_bsTCUState/1 -> Bus Selector/1
  Bus Selector/1 -> Compare To Constant/1  "<TCU_ActualGear>"
  Compare To Constant/1 -> GearEC_stGearECFlg/1

== system LKAS_AutoSave_20210315_1628/LKAS/LL/LLOn/LL State Determination (LLStateDet)/LL State Machine Conditions (LLSMCon)/Enable Condition (EnaC)/Vehicle State Condition (VehStateC)/Vehicle Speed Enable Condition (VehSpdEC) ==
  VehSpdEC_stDACMode : Inport
  VehSpdEC_vVehSpd : Inport  Port=2
  VehSpdEC_vLDWVehSpdMax_C : Inport  Port=3
  VehSpdEC_vLKAVehSpdMax_C : Inport  Port=4
  VehSpdEC_vVehSpdMin_C : Inport  Port=5
  Interval Test Dynamic : simulink/Logic and Bit Operations/Interval Test Dynamic  IntervalClosedRight=on  IntervalClosedLeft=on  OutDataTypeStr=boolean
      settings: SourceProductName=Simulink  SourceProductBaseCode=SL
  Switch : Switch  Threshold=2
  VehSpdEC_stVehSpdECFlg : Outport
  wires:
  VehSpdEC_vVehSpd/1 -> Interval Test Dynamic/2
  VehSpdEC_vVehSpdMin_C/1 -> Interval Test Dynamic/3
  Interval Test Dynamic/1 -> VehSpdEC_stVehSpdECFlg/1
  VehSpdEC_stDACMode/1 -> Switch/2
  VehSpdEC_vLKAVehSpdMax_C/1 -> Switch/1
  Switch/1 -> Interval Test Dynamic/1
  VehSpdEC_vLDWVehSpdMax_C/1 -> Switch/3

== system LKAS_AutoSave_20210315_1628/LKAS/LL/LLOn/LL State Determination (LLStateDet)/LL State Machine Conditions (LLSMCon)/Enable Condition (EnaC)/Vehicle State Condition (VehStateC)/Vehicle State Condition Synthesis (VehStateCSyn) ==
  VehStateCSyn_stVehSpdECFlg : Inport
  VehStateCSyn_stEmgcyLghtECFlg : Inport  Port=2
  VehStateCSyn_stGearECFlg : Inport  Port=3
  Logical Operator : Logic  Inputs=3  AllPortsSameDT=off  OutDataTypeStr=boolean
  VehStateCSyn_stVehStateCSyn : Outport
  wires:
  VehStateCSyn_stVehSpdECFlg/1 -> Logical Operator/1
  VehStateCSyn_stGearECFlg/1 -> Logical Operator/3
  Logical Operator/1 -> VehStateCSyn_stVehStateCSyn/1
  VehStateCSyn_stEmgcyLghtECFlg/1 -> Logical Operator/2

== system LKAS_AutoSave_20210315_1628/LKAS/LL/LLOn/LKA/LKA Motion Planning (LKAMP) /Switching Condition (SwtCon)/Ending Heading Angle Determination (EndHdAgDet)/Lateral Speed Compensation (LSpdComp)/If Action Subsystem ==
  In1 : Inport
  Action Port : ActionPort  InitializeStates=reset  ActionType=then
      settings: AttributesFormatString=states = %<InitializeStates>
  Cast To Single1 : DataTypeConversion  LockScale=on
  Out1 : Outport  InitialOutput=0
      settings: AttributesFormatString=%<OutputWhenDisabled> = %<InitialOutput>
  wires:
  Cast To Single1/1 -> Out1/1
  In1/1 -> Cast To Single1/1

== system LKAS_AutoSave_20210315_1628/LKAS/LL/LLOn/LKA/LKA Motion Planning (LKAMP) /Switching Condition (SwtCon)/Ending Heading Angle Determination (EndHdAgDet)/Lateral Speed Compensation (LSpdComp)/If Action Subsystem2 ==
  Action Port : ActionPort  InitializeStates=reset  ActionType=else
      settings: AttributesFormatString=states = %<InitializeStates>
  Constant : Constant  Value=0  OutDataTypeStr=single
  Out1 : Outport  InitialOutput=0
      settings: AttributesFormatString=%<OutputWhenDisabled> = %<InitialOutput>
  wires:
  Constant/1 -> Out1/1

== system LKAS_AutoSave_20210315_1628/LKAS/LL/LLOn/LKA/LKA Motion Planning (LKAMP) /Switching Condition (SwtCon)/Ending Heading Angle Determination (EndHdAgDet)/Lateral Speed Compensation (LSpdComp)/If Action Subsystem4 ==
  In1 : Inport
  Action Port : ActionPort  InitializeStates=reset  ActionType=elseif
      settings: AttributesFormatString=states = %<InitializeStates>
  Cast To Single1 : DataTypeConversion  LockScale=on
  Out1 : Outport  InitialOutput=0
      settings: AttributesFormatString=%<OutputWhenDisabled> = %<InitialOutput>
  wires:
  Cast To Single1/1 -> Out1/1
  In1/1 -> Cast To Single1/1

== system LKAS_AutoSave_20210315_1628/LKAS/LL/LLOn/LKA/Lane Following (LF)/Trajectory Following Control (TFC)/Feedback Control (FbCtl)/Subsystem/If Action Subsystem ==
  In1 : Inport
  Action Port : ActionPort  ActionType=then
      settings: AttributesFormatString=states = %<InitializeStates>
  Out1 : Outport
      settings: AttributesFormatString=%<OutputWhenDisabled> = %<InitialOutput>
  wires:
  In1/1 -> Out1/1

== system LKAS_AutoSave_20210315_1628/LKAS/LL/LLOn/LKA/Lane Following (LF)/Trajectory Following Control (TFC)/Feedback Control (FbCtl)/Subsystem/If Action Subsystem1 ==
  In1 : Inport
  Action Port : ActionPort  ActionType=elseif
      settings: AttributesFormatString=states = %<InitializeStates>
  Out1 : Outport
      settings: AttributesFormatString=%<OutputWhenDisabled> = %<InitialOutput>
  wires:
  In1/1 -> Out1/1

== system LKAS_AutoSave_20210315_1628/LKAS/LL/LLOn/LKA/Lane Following (LF)/Trajectory Following Control (TFC)/Feedback Control (FbCtl)/Subsystem/If Action Subsystem2 ==
  In1 : Inport
  Action Port : ActionPort  ActionType=else
      settings: AttributesFormatString=states = %<InitializeStates>
  Out1 : Outport
      settings: AttributesFormatString=%<OutputWhenDisabled> = %<InitialOutput>
  wires:
  In1/1 -> Out1/1

== system LKAS_AutoSave_20210315_1628/LKAS/LL/LLOn/LKA/Lane Following (LF)/Trajectory Following Control (TFC)/Feedback Control (FbCtl)/Subsystem/Signal Latching2 ==
  In : Inport
  Add : Sum  OutDataTypeStr=uint16
  Constant : Constant  OutDataTypeStr=uint16  SampleTime=-1
  Constant2 : Constant  Value=LatchTime  OutDataTypeStr=uint16  SampleTime=-1
  If : If  NumInputs=2  IfExpression=u1==u2  ShowElse=off
  Memory : Memory  InheritSampleTime=on
  Saturation1 : Saturate  UpperLimit=10000  LowerLimit=0  OutDataTypeStr=uint16
  "if action " : Subsystem  TreatAsAtomicUnit=on
  Out : Outport
  wires:
  Constant2/1 -> If/2
  In/1 -> "if action "/1(In)
  "if action "/1(Out) -> Out/1
  If/1 -> "if action "/Action
  Constant/1 -> Add/1
  Add/1 -> Saturation1/1
  Memory/1 -> Add/2
  Saturation1/1 -> Memory/1, If/1

== system LKAS_AutoSave_20210315_1628/LKAS/LL/LLOn/LKA/Plan To LaneFollowing (PTLF)/InsideJudge1/If Action Subsystem/If Action Subsystem/Signal Latching ==
  In : Inport
  Add : Sum  OutDataTypeStr=uint16
  Constant : Constant  OutDataTypeStr=uint16  SampleTime=-1
  Constant2 : Constant  Value=LatchTime  OutDataTypeStr=uint16  SampleTime=-1
  If : If  NumInputs=2  IfExpression=u1<=u2  ShowElse=off
  Memory : Memory  InheritSampleTime=on
  Saturation1 : Saturate  UpperLimit=10000  LowerLimit=0  OutDataTypeStr=uint16
  "if action " : Subsystem  TreatAsAtomicUnit=on
  Out : Outport
  wires:
  Saturation1/1 -> If/1, Memory/1
  Memory/1 -> Add/2
  Add/1 -> Saturation1/1
  Constant/1 -> Add/1
  If/1 -> "if action "/Action
  "if action "/1(Out) -> Out/1
  In/1 -> "if action "/1(In)
  Constant2/1 -> If/2

== system LKAS_AutoSave_20210315_1628/LKAS/LL/LLOn/LKA/Plan To LaneFollowing (PTLF)/InsideJudge1/If Action Subsystem/If Action Subsystem/Signal Latching1 ==
  In : Inport
  Add : Sum  OutDataTypeStr=uint16
  Constant : Constant  OutDataTypeStr=uint16  SampleTime=-1
  Constant2 : Constant  Value=LatchTime  OutDataTypeStr=uint16  SampleTime=-1
  If : If  NumInputs=2  IfExpression=u1==u2  ShowElse=off
  Memory : Memory  InheritSampleTime=on
  Saturation1 : Saturate  UpperLimit=10000  LowerLimit=0  OutDataTypeStr=uint16
  "if action " : Subsystem  TreatAsAtomicUnit=on
  Out : Outport
  wires:
  Constant2/1 -> If/2
  In/1 -> "if action "/1(In)
  "if action "/1(Out) -> Out/1
  If/1 -> "if action "/Action
  Constant/1 -> Add/1
  Add/1 -> Saturation1/1
  Memory/1 -> Add/2
  Saturation1/1 -> Memory/1, If/1

== system LKAS_AutoSave_20210315_1628/LKAS/LL/LLOn/LKA/Plan To LaneFollowing (PTLF)/InsideJudge1/If Action Subsystem1/If Action Subsystem/Signal Latching ==
  In : Inport
  Add : Sum  OutDataTypeStr=uint16
  Constant : Constant  OutDataTypeStr=uint16  SampleTime=-1
  Constant2 : Constant  Value=LatchTime  OutDataTypeStr=uint16  SampleTime=-1
  If : If  NumInputs=2  IfExpression=u1<=u2  ShowElse=off
  Memory : Memory  InheritSampleTime=on
  Saturation1 : Saturate  UpperLimit=10000  LowerLimit=0  OutDataTypeStr=uint16
  "if action " : Subsystem  TreatAsAtomicUnit=on
  Out : Outport
  wires:
  Saturation1/1 -> If/1, Memory/1
  Memory/1 -> Add/2
  Add/1 -> Saturation1/1
  Constant/1 -> Add/1
  If/1 -> "if action "/Action
  "if action "/1(Out) -> Out/1
  In/1 -> "if action "/1(In)
  Constant2/1 -> If/2

== system LKAS_AutoSave_20210315_1628/LKAS/LL/LLOn/LKA/Plan To LaneFollowing (PTLF)/InsideJudge1/If Action Subsystem1/If Action Subsystem/Signal Latching1 ==
  In : Inport
  Add : Sum  OutDataTypeStr=uint16
  Constant : Constant  OutDataTypeStr=uint16  SampleTime=-1
  Constant2 : Constant  Value=LatchTime  OutDataTypeStr=uint16  SampleTime=-1
  If : If  NumInputs=2  IfExpression=u1==u2  ShowElse=off
  Memory : Memory  InheritSampleTime=on
  Saturation1 : Saturate  UpperLimit=10000  LowerLimit=0  OutDataTypeStr=uint16
  "if action " : Subsystem  TreatAsAtomicUnit=on
  Out : Outport
  wires:
  Constant2/1 -> If/2
  In/1 -> "if action "/1(In)
  "if action "/1(Out) -> Out/1
  If/1 -> "if action "/Action
  Constant/1 -> Add/1
  Add/1 -> Saturation1/1
  Memory/1 -> Add/2
  Saturation1/1 -> Memory/1, If/1

== system LKAS_AutoSave_20210315_1628/LKAS/LL/LLOn/LL State Determination (LLStateDet)/LL State Machine Conditions (LLSMCon)/Activation Condition (ActvC)/Deviation Threshold Condition (DvtThresCon)/Deviation Threshold Judgement LDW (DvtThresJdg)/Deviation Speed Detection (DvtSpdDet) ==
  DvtSpdDet_vLftDvtSpd : Inport
  DvtSpdDet_vRgtDvtSpd : Inport  Port=2
  DvtSpdDet_vDvtSpdMin_C : Inport  Port=3
  If : If  NumInputs=3  IfExpression=u1>=u3 & u2>=u3  ElseIfExpressions=u1<=-u3 & u2<=-u3
  Memory : Memory  InheritSampleTime=on
  Merge1 : Merge  Inputs=3
  Ph1SWA : Subsystem
  Ph2SWA : Subsystem
  Ph3SWA : Subsystem
  DvtSpdDet_stDvtSpdFlg : Outport
  wires:
  Memory/1 -> Ph3SWA/1(In1)
  Merge1/1 -> DvtSpdDet_stDvtSpdFlg/1, Memory/1
  If/3 -> Ph3SWA/Action
  If/2 -> Ph2SWA/Action
  Ph3SWA/1(Out) -> Merge1/3
  Ph2SWA/1(Out) -> Merge1/2
  Ph1SWA/1(Out) -> Merge1/1
  If/1 -> Ph1SWA/Action
  DvtSpdDet_vDvtSpdMin_C/1 -> If/3
  DvtSpdDet_vRgtDvtSpd/1 -> If/2
  DvtSpdDet_vLftDvtSpd/1 -> If/1

== system LKAS_AutoSave_20210315_1628/LKAS/LL/LLOn/LL State Determination (LLStateDet)/LL State Machine Conditions (LLSMCon)/Activation Condition (ActvC)/Deviation Threshold Condition (DvtThresCon)/Deviation Threshold Judgement LDW (DvtThresJdg)/Deviation Threshold Condition Synthesis (DTCSyn) ==
  DTCSyn_stLftDvtThresActvFlg : Inport
  DTCSyn_stRgtDvtThresActvFlg : Inport  Port=2
  DTCSyn_stDvtSpdFlg : Inport  Port=3
  Cast To Single : DataTypeConversion  OutDataTypeStr=uint8
  Cast To Single1 : DataTypeConversion  OutDataTypeStr=uint8
  Cast To Single2 : DataTypeConversion  LockScale=on
  Constant2 : Constant  Value=0  OutDataTypeStr=uint8
  Gain1 : Gain  Gain=2  OutDataTypeStr=Inherit: Same as input
  Switch2 : Switch  Criteria=u2 > Threshold
  Switch3 : Switch
  DTCSyn_stDvtThresActvFlg : Outport
  wires:
  Cast To Single1/1 -> Gain1/1
  Cast To Single/1 -> Cast To Single2/1
  Gain1/1 -> Switch3/3  "DvtThresActvFlg"
  Cast To Single2/1 -> Switch2/1  "DvtThresActvFlg"
  Constant2/1 -> Switch2/3  "DvtThresActvFlg"
  DTCSyn_stDvtSpdFlg/1 -> Switch2/2, Switch3/2
  Switch3/1 -> DTCSyn_stDvtThresActvFlg/1
  Switch2/1 -> Switch3/1
  DTCSyn_stLftDvtThresActvFlg/1 -> Cast To Single/1
  DTCSyn_stRgtDvtThresActvFlg/1 -> Cast To Single1/1

== system LKAS_AutoSave_20210315_1628/LKAS/LL/LLOn/LL State Determination (LLStateDet)/LL State Machine Conditions (LLSMCon)/Activation Condition (ActvC)/Deviation Threshold Condition (DvtThresCon)/Deviation Threshold Judgement LDW (DvtThresJdg)/Left Side Deviation Threshold Condition (LftDTC) ==
  LftDTC_bsDvtThresInfo : Inport
  LftDTC_lLftDvt : Inport  Port=2
  LftDTC_vLftDvtSpd : Inport  Port=3
  Abs : Abs
  Bus Selector : BusSelector  OutputSignals=LL_ThresDet_lDvtThresLwrLDW,LL_ThresDet_lDvtThresUprLDW,LL_ThresDet_tiTTLCThresLDW
  Divide : Product  Inputs=**
  Relational Operator2 : RelationalOperator  Operator=<=  OutDataTypeStr=boolean  RndMeth=Nearest
  Saturation Dynamic : simulink/Discontinuities/Saturation Dynamic  OutMin=[]  OutMax=[]  OutDataTypeStr=Inherit: Same as second input  OutDataType=fixdt(1, 16)  OutScaling=2^-10  DoSatur=off
  LftDTC_stLftDvtThresActvFlg : Outport
  wires:
  Abs/1 -> Divide/2
  Saturation Dynamic/1 -> Relational Operator2/2
  Divide/1 -> Saturation Dynamic/2
  LftDTC_vLftDvtSpd/1 -> Abs/1
  LftDTC_lLftDvt/1 -> Relational Operator2/1
  Relational Operator2/1 -> LftDTC_stLftDvtThresActvFlg/1
  Bus Selector/2 -> Saturation Dynamic/1  "<LL_ThresDet_lDvtThresUprLDW>"
  Bus Selector/3 -> Divide/1  "<LL_ThresDet_tiTTLCThresLDW>"
  Bus Selector/1 -> Saturation Dynamic/3  "<LL_ThresDet_lDvtThresLwrLDW>"
  LftDTC_bsDvtThresInfo/1 -> Bus Selector/1

== system LKAS_AutoSave_20210315_1628/LKAS/LL/LLOn/LL State Determination (LLStateDet)/LL State Machine Conditions (LLSMCon)/Activation Condition (ActvC)/Deviation Threshold Condition (DvtThresCon)/Deviation Threshold Judgement LDW (DvtThresJdg)/Right Side Deviation Threshold Condition (RgtDTC) ==
  RgtDTC_bsDvtThresInfo : Inport
  RgtDTC_lRgtDvt : Inport  Port=2
  RgtDTC_vRgtDvtSpd : Inport  Port=3
  Abs : Abs
  Bus Selector : BusSelector  OutputSignals=LL_ThresDet_lDvtThresLwrLDW,LL_ThresDet_lDvtThresUprLDW,LL_ThresDet_tiTTLCThresLDW
  Divide : Product  Inputs=**
  Relational Operator2 : RelationalOperator  Operator=<=  OutDataTypeStr=boolean  RndMeth=Nearest
  Saturation Dynamic : simulink/Discontinuities/Saturation Dynamic  OutMin=[]  OutMax=[]  OutDataTypeStr=Inherit: Same as second input  OutDataType=fixdt(1, 16)  OutScaling=2^-10  DoSatur=off
  RgtDTC_stRgtDvtThresActvFlg : Outport
  wires:
  Bus Selector/3 -> Divide/1  "<LL_ThresDet_tiTTLCThresLDW>"
  Bus Selector/2 -> Saturation Dynamic/1  "<LL_ThresDet_lDvtThresUprLDW>"
  Bus Selector/1 -> Saturation Dynamic/3  "<LL_ThresDet_lDvtThresLwrLDW>"
  RgtDTC_vRgtDvtSpd/1 -> Abs/1
  Saturation Dynamic/1 -> Relational Operator2/2
  Divide/1 -> Saturation Dynamic/2
  Abs/1 -> Divide/2
  RgtDTC_lRgtDvt/1 -> Relational Operator2/1
  Relational Operator2/1 -> RgtDTC_stRgtDvtThresActvFlg/1
  RgtDTC_bsDvtThresInfo/1 -> Bus Selector/1

== system LKAS_AutoSave_20210315_1628/LKAS/LL/LLOn/LL State Determination (LLStateDet)/LL State Machine Conditions (LLSMCon)/Activation Condition (ActvC)/Deviation Threshold Condition (DvtThresCon)/Deviation Threshold Judgement LKA (DvtThresJdg)/Deviation Speed Detection (DvtSpdDet) ==
  DvtSpdDet_vLftDvtSpd : Inport
  DvtSpdDet_vRgtDvtSpd : Inport  Port=2
  DvtSpdDet_vDvtSpdMin_C : Inport  Port=3
  If : If  NumInputs=3  IfExpression=u1>=u3 & u2>=u3  ElseIfExpressions=u1<=-u3 & u2<=-u3
  Merge1 : Merge  Inputs=3
  Ph1SWA : Subsystem
  Ph2SWA : Subsystem
  Ph3SWA : Subsystem
  DvtSpdDet_stDvtSpdFlg : Outport
  wires:
  DvtSpdDet_vLftDvtSpd/1 -> If/1
  DvtSpdDet_vRgtDvtSpd/1 -> If/2
  DvtSpdDet_vDvtSpdMin_C/1 -> If/3
  If/1 -> Ph1SWA/Action
  Ph1SWA/1(Out) -> Merge1/1
  Ph2SWA/1(Out) -> Merge1/2
  Ph3SWA/1(Out) -> Merge1/3
  If/2 -> Ph2SWA/Action
  If/3 -> Ph3SWA/Action
  Merge1/1 -> DvtSpdDet_stDvtSpdFlg/1

== system LKAS_AutoSave_20210315_1628/LKAS/LL/LLOn/LL State Determination (LLStateDet)/LL State Machine Conditions (LLSMCon)/Activation Condition (ActvC)/Deviation Threshold Condition (DvtThresCon)/Deviation Threshold Judgement LKA (DvtThresJdg)/Deviation Threshold Condition Synthesis (DTCSyn) ==
  DTCSyn_stLftDvtThresActvFlg : Inport
  DTCSyn_stRgtDvtThresActvFlg : Inport  Port=2
  DTCSyn_stDvtSpdFlg : Inport  Port=3
  Cast To Single : DataTypeConversion  OutDataTypeStr=uint8
  Cast To Single1 : DataTypeConversion  OutDataTypeStr=uint8
  Constant2 : Constant  Value=0  OutDataTypeStr=uint8
  Gain1 : Gain  Gain=2  OutDataTypeStr=Inherit: Same as input
  Switch2 : Switch  Criteria=u2 > Threshold
  Switch3 : Switch
  DTCSyn_stDvtThresActvFlg : Outport
  wires:
  Cast To Single1/1 -> Gain1/1
  Switch2/1 -> Switch3/1
  Switch3/1 -> DTCSyn_stDvtThresActvFlg/1
  Constant2/1 -> Switch2/3  "DvtThresActvFlg"
  DTCSyn_stDvtSpdFlg/1 -> Switch2/2, Switch3/2
  Cast To Single/1 -> Switch2/1  "DvtThresActvFlg"
  Gain1/1 -> Switch3/3  "DvtThresActvFlg"
  DTCSyn_stLftDvtThresActvFlg/1 -> Cast To Single/1
  DTCSyn_stRgtDvtThresActvFlg/1 -> Cast To Single1/1

== system LKAS_AutoSave_20210315_1628/LKAS/LL/LLOn/LL State Determination (LLStateDet)/LL State Machine Conditions (LLSMCon)/Activation Condition (ActvC)/Deviation Threshold Condition (DvtThresCon)/Deviation Threshold Judgement LKA (DvtThresJdg)/Left Side Deviation Threshold Condition (LftDTC) ==
  LftDTC_bsDvtThresInfo : Inport
  LftDTC_lLftDvt : Inport  Port=2
  LftDTC_vLftDvtSpd : Inport  Port=3
  Abs : Abs
  Bus Selector : BusSelector  OutputSignals=LL_ThresDet_lDvtThresLwrLKA,LL_ThresDet_lDvtThresUprLKA,LL_ThresDet_tiTTLCThresLKA
  Constant : Constant  Value=0  OutDataTypeStr=single
  Divide : Product  Inputs=**
  Logical Operator : Logic  AllPortsSameDT=off  OutDataTypeStr=boolean
  Relational Operator1 : RelationalOperator  Operator=<  OutDataTypeStr=boolean  RndMeth=Nearest
  Relational Operator3 : RelationalOperator  Operator=<=  OutDataTypeStr=boolean  RndMeth=Nearest
  Saturation Dynamic : simulink/Discontinuities/Saturation Dynamic  OutMin=[]  OutMax=[]  OutDataTypeStr=Inherit: Same as second input  OutDataType=fixdt(1, 16)  OutScaling=2^-10  DoSatur=off
  LftDTC_stLftDvtThresActvFlg : Outport
  wires:
  LftDTC_bsDvtThresInfo/1 -> Bus Selector/1
  Bus Selector/1 -> Saturation Dynamic/3  "<LL_ThresDet_lDvtThresLwrLKA>"
  Bus Selector/3 -> Divide/1  "<LL_ThresDet_tiTTLCThresLKA>"
  Bus Selector/2 -> Saturation Dynamic/1  "<LL_ThresDet_lDvtThresUprLKA>"
  Relational Operator3/1 -> Logical Operator/2
  LftDTC_lLftDvt/1 -> Relational Operator1/2, Relational Operator3/1
  LftDTC_vLftDvtSpd/1 -> Abs/1
  Divide/1 -> Saturation Dynamic/2
  Saturation Dynamic/1 -> Relational Operator3/2
  Abs/1 -> Divide/2
  Logical Operator/1 -> LftDTC_stLftDvtThresActvFlg/1
  Constant/1 -> Relational Operator1/1
  Relational Operator1/1 -> Logical Operator/1

== system LKAS_AutoSave_20210315_1628/LKAS/LL/LLOn/LL State Determination (LLStateDet)/LL State Machine Conditions (LLSMCon)/Activation Condition (ActvC)/Deviation Threshold Condition (DvtThresCon)/Deviation Threshold Judgement LKA (DvtThresJdg)/Right Side Deviation Threshold Condition (RgtDTC) ==
  RgtDTC_bsDvtThresInfo : Inport
  RgtDTC_lRgtDvt : Inport  Port=2
  RgtDTC_vRgtDvtSpd : Inport  Port=3
  Abs : Abs
  Bus Selector : BusSelector  OutputSignals=LL_ThresDet_lDvtThresLwrLKA,LL_ThresDet_lDvtThresUprLKA,LL_ThresDet_tiTTLCThresLKA
  Constant : Constant  Value=0  OutDataTypeStr=single
  Divide : Product  Inputs=**
  Logical Operator : Logic  AllPortsSameDT=off  OutDataTypeStr=boolean
  Relational Operator1 : RelationalOperator  Operator=<  OutDataTypeStr=boolean  RndMeth=Nearest
  Relational Operator2 : RelationalOperator  Operator=<=  OutDataTypeStr=boolean  RndMeth=Nearest
  Saturation Dynamic : simulink/Discontinuities/Saturation Dynamic  OutMin=[]  OutMax=[]  OutDataTypeStr=Inherit: Same as second input  OutDataType=fixdt(1, 16)  OutScaling=2^-10  DoSatur=off
  RgtDTC_stRgtDvtThresActvFlg : Outport
  wires:
  Abs/1 -> Divide/2
  RgtDTC_bsDvtThresInfo/1 -> Bus Selector/1
  Relational Operator2/1 -> Logical Operator/2
  RgtDTC_vRgtDvtSpd/1 -> Abs/1
  Divide/1 -> Saturation Dynamic/2
  Saturation Dynamic/1 -> Relational Operator2/2
  Bus Selector/1 -> Saturation Dynamic/3  "<LL_ThresDet_lDvtThresLwrLKA>"
  Bus Selector/2 -> Saturation Dynamic/1  "<LL_ThresDet_lDvtThresUprLKA>"
  Bus Selector/3 -> Divide/1  "<LL_ThresDet_tiTTLCThresLKA>"
  Constant/1 -> Relational Operator1/1
  Relational Operator1/1 -> Logical Operator/1
  RgtDTC_lRgtDvt/1 -> Relational Operator1/2, Relational Operator2/1
  Logical Operator/1 -> RgtDTC_stRgtDvtThresActvFlg/1

== system LKAS_AutoSave_20210315_1628/LKAS/LL/LLOn/LL State Determination (LLStateDet)/LL State Machine Conditions (LLSMCon)/Deactivation Condition (DeactvC)/Deviation Threshold Condition (DvtThresCon)/Deviation Threshold Judgement LDW (DvtThresJdg)/Deviation Speed Detection (DvtSpdDet) ==
  DvtSpdDet_vLftDvtSpd : Inport
  DvtSpdDet_vRgtDvtSpd : Inport  Port=2
  DvtSpdDet_vDvtSpdMin_C : Inport  Port=3
  If : If  NumInputs=3  IfExpression=u1>=u3 & u2>=u3  ElseIfExpressions=u1<=-u3 & u2<=-u3
  Memory : Memory  InheritSampleTime=on
  Merge1 : Merge  Inputs=3
  Ph1SWA : Subsystem
  Ph2SWA : Subsystem
  Ph3SWA : Subsystem
  DvtSpdDet_stDvtSpdFlg : Outport
  wires:
  Memory/1 -> Ph3SWA/1(In1)
  Merge1/1 -> DvtSpdDet_stDvtSpdFlg/1, Memory/1
  If/3 -> Ph3SWA/Action
  If/2 -> Ph2SWA/Action
  Ph3SWA/1(Out) -> Merge1/3
  Ph2SWA/1(Out) -> Merge1/2
  Ph1SWA/1(Out) -> Merge1/1
  If/1 -> Ph1SWA/Action
  DvtSpdDet_vDvtSpdMin_C/1 -> If/3
  DvtSpdDet_vRgtDvtSpd/1 -> If/2
  DvtSpdDet_vLftDvtSpd/1 -> If/1

== system LKAS_AutoSave_20210315_1628/LKAS/LL/LLOn/LL State Determination (LLStateDet)/LL State Machine Conditions (LLSMCon)/Deactivation Condition (DeactvC)/Deviation Threshold Condition (DvtThresCon)/Deviation Threshold Judgement LDW (DvtThresJdg)/Deviation Threshold Condition Synthesis (DTCSyn) ==
  DTCSyn_stLftDvtThresActvFlg : Inport
  DTCSyn_stRgtDvtThresActvFlg : Inport  Port=2
  DTCSyn_stDvtSpdFlg : Inport  Port=3
  Cast To Single : DataTypeConversion  OutDataTypeStr=uint8
  Cast To Single1 : DataTypeConversion  OutDataTypeStr=uint8
  Cast To Single2 : DataTypeConversion  LockScale=on
  Constant2 : Constant  Value=0  OutDataTypeStr=uint8
  Gain1 : Gain  Gain=2  OutDataTypeStr=Inherit: Same as input
  Switch2 : Switch  Criteria=u2 > Threshold
  Switch3 : Switch
  DTCSyn_stDvtThresActvFlg : Outport
  wires:
  Cast To Single1/1 -> Gain1/1
  Cast To Single/1 -> Cast To Single2/1
  Gain1/1 -> Switch3/3  "DvtThresActvFlg"
  Cast To Single2/1 -> Switch2/1  "DvtThresActvFlg"
  Constant2/1 -> Switch2/3  "DvtThresActvFlg"
  DTCSyn_stDvtSpdFlg/1 -> Switch2/2, Switch3/2
  Switch3/1 -> DTCSyn_stDvtThresActvFlg/1
  Switch2/1 -> Switch3/1
  DTCSyn_stLftDvtThresActvFlg/1 -> Cast To Single/1
  DTCSyn_stRgtDvtThresActvFlg/1 -> Cast To Single1/1

== system LKAS_AutoSave_20210315_1628/LKAS/LL/LLOn/LL State Determination (LLStateDet)/LL State Machine Conditions (LLSMCon)/Deactivation Condition (DeactvC)/Deviation Threshold Condition (DvtThresCon)/Deviation Threshold Judgement LDW (DvtThresJdg)/Left Side Deviation Threshold Condition (LftDTC) ==
  LftDTC_bsDvtThresInfo : Inport
  LftDTC_lLftDvt : Inport  Port=2
  LftDTC_vLftDvtSpd : Inport  Port=3
  Abs : Abs
  Bus Selector : BusSelector  OutputSignals=LL_ThresDet_lDvtThresLwrLDW,LL_ThresDet_lDvtThresUprLDW,LL_ThresDet_tiTTLCThresLDW
  Divide : Product  Inputs=**
  Relational Operator2 : RelationalOperator  Operator=<=  OutDataTypeStr=boolean  RndMeth=Nearest
  Saturation Dynamic : simulink/Discontinuities/Saturation Dynamic  OutMin=[]  OutMax=[]  OutDataTypeStr=Inherit: Same as second input  OutDataType=fixdt(1, 16)  OutScaling=2^-10  DoSatur=off
  LftDTC_stLftDvtThresActvFlg : Outport
  wires:
  Abs/1 -> Divide/2
  Saturation Dynamic/1 -> Relational Operator2/2
  Divide/1 -> Saturation Dynamic/2
  LftDTC_vLftDvtSpd/1 -> Abs/1
  LftDTC_lLftDvt/1 -> Relational Operator2/1
  Relational Operator2/1 -> LftDTC_stLftDvtThresActvFlg/1
  Bus Selector/2 -> Saturation Dynamic/1  "<LL_ThresDet_lDvtThresUprLDW>"
  Bus Selector/3 -> Divide/1  "<LL_ThresDet_tiTTLCThresLDW>"
  Bus Selector/1 -> Saturation Dynamic/3  "<LL_ThresDet_lDvtThresLwrLDW>"
  LftDTC_bsDvtThresInfo/1 -> Bus Selector/1
